simulink library "simulink"  (Simulink 6.0)
settings: Solver=ode45  SolverMode=SingleTasking  StartTime=0.0  StopTime=10.0  RelTol=1e-3
PostLoadFcn:
  | setsysloc(bdroot)
undefined symbols (not defined in the file or in its folder): DiscIntNeverNeededParam, getdatatypespecs, NumBits1, NumBits2, sfunxy, sigbuilder_block, slcm, Slope1, Slope2
libraries: simulink x82, eml_lib x1
(part 1 of 5)
settings Model: RequirementInfo=9  CovMetricSettings=d  Creator=ricks  LastModifiedBy=dyang  ExtModeAutoUpdateStatusClock=off  ProdHWDeviceType=Specified
settings Model: ForwardingTableString=|
  | ||__slOldName__||simulink/Discrete/Additional
  | Transfer Fcns/Weighted
  | Moving Average||__slNewName__||simulink/Discrete/Weighted
  | Moving Average||__slOldName__||simulink/Discrete/Additional
  | Transfer Fcns/Transfer Fcn
  | Direct Form I||__slNewName__||fixpt_lib_4/Filters/Filter
  | Direct Form I||__slOldName__||simulink/Bit
  | Operations/Bitwise
  | Operator||__slNewName__||simulink/Logic and Bit
  | Operations/Bitwise
  | Operator||__slOldName__||simulink/Logic and Bit
  | Operations/Bitwise
  | Logical Operator||__slNewName__||simulink/Logic and Bit
  | Operations/Bitwise
  | Operator||__slOldName__||simulink/Math
  | Operations/Bitwise
  | Logical Operator||__slNewName__||simulink/Logic and Bit
  | Operations/Bitwise
  | Operator||__slOldName__||simulink/Look-Up
  | Tables/Direct Look-Up
  | Table (n-D)||__slNewName__||simulink/Lookup
  | Tables/Direct Lookup
  | Table (n-D)||__slOldName__||simulink/Look-Up
  | Tables/Interpolation (n-D)
  | using PreLook-Up||__slNewName__||simulink/Lookup
  | Tables/Interpolation (n-D)
  | using PreLookup||__slOldName__||simulink/Look-Up
  | Tables/PreLook-Up
  | Index Search||__slNewName__||simulink/Lookup
  | Tables/PreLookup
  | Index Search||__slOldName__||simulink/Look-Up
  | Tables/Look-Up
  | Table (n-D)||__slNewName__||simulink/Lookup
  | Tables/Lookup
  | Table (n-D)||__slOldName__||simulink/Linear/Matrix
  | Gain||__slNewName__||simulink3/Math/Matrix
  | Gain||__slOldName__||simulink/Connections/Model Info||__slNewName__||simulink/Model-Wide
  | Utilities/Model Info||__slOldName__||simulink/Nonlinear/Manual Switch||__slNewName__||simulink/Signal
  | Routing/Manual Switch||__slOldName__||simulink/Nonlinear/Coulomb &
  | Viscous Friction||__slNewName__||simulink/Discontinuities/Coulomb &
  | Viscous Friction||__slOldName__||simulink/Linear/Slider
  | Gain||__slNewName__||simulink/Math
  | Operations/Slider
  | Gain||__slOldName__||simulink/Nonlinear/Algebraic Constraint||__slNewName__||simulink/Math
  | Operations/Algebraic Constraint||__slOldName__||simulink/Nonlinear/Look-Up
  | Table (2-D)||__slNewName__||simulink/Lookup
  | Tables/Lookup
  | Table (2-D)||__slOldName__||simulink/Linear/Dot Product||__slNewName__||simulink/Math
  | Operations/Dot Product
settings DataIOCC: SignalLoggingName=logsOut
settings OptimizationCC: BooleanDataType=off
settings DebuggingCC: CheckExecutionContextPreStartOutputMsg=on  CheckExecutionContextRuntimeOutputMsg=on  SolverPrmCheckMsg=none
settings HardwareCC: ProdHWDeviceType=Specified  TargetUnknown=on
settings ModelReferenceCC: UpdateModelReferenceTargets=IfOutOfDate

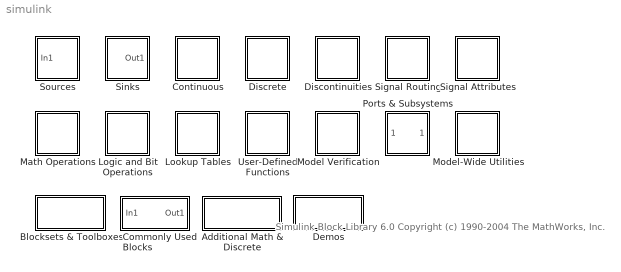
== system simulink ==
  note: Simulink Block Library 6.0
      | Copyright (c) 1990-2004
      | The MathWorks, Inc.
  Additional Math & Discrete : Subsystem
      mask Display: image(imread('additional_math_discrete.bmp','bmp'))
  Blocksets & Toolboxes : Subsystem
      settings: OpenFcn=findblib
      mask Display: image(imread('blocksets.bmp','bmp'))
  Commonly Used Blocks : Subsystem
      mask Display: image(imread('commonly_used.bmp','bmp'))
  Continuous : Subsystem
      mask Display: image(imread('continuous.bmp','bmp'))
  Demos : Subsystem
      settings: OpenFcn=demo simulink
      mask Display: image(imread('demos.bmp','bmp'))
  Discontinuities : Subsystem
      mask Display: image(imread('nonlinear.bmp','bmp'))
  Discrete : Subsystem
      mask Display: image(imread('discrete.bmp','bmp'))
  Logic and Bit Operations : Subsystem
      mask Display: image(imread('logical_bit.bmp','bmp'))
  Lookup Tables : Subsystem
      mask Display: image(imread('tables.bmp','bmp'))
  Math Operations : Subsystem
      mask Display: image(imread('math.bmp','bmp'))
  Model Verification : Subsystem
      mask Display: image(imread('assertion.bmp','bmp'))
  Model-Wide Utilities : Subsystem
      mask Display: image(imread('misc.bmp','bmp'))
  Ports & Subsystems : Subsystem  TreatAsAtomicUnit=on
      mask Display: image(imread('subsystems.bmp','bmp'))
  Signal Attributes : Subsystem
      mask Display: image(imread('attributes.bmp','bmp'))
  Signal Routing : Subsystem
      mask Display: image(imread('signals.bmp','bmp'))
  Sinks : Subsystem
      mask Display: image(imread('sinks.bmp','bmp'))
  Sources : Subsystem
      mask Display: image(imread('sources.bmp','bmp'))
  User-Defined Functions : Subsystem
      mask Display: image(imread('functions.bmp','bmp'))

== system simulink/Additional Math & Discrete ==
  note: Additional Math & Discrete
  Additional Discrete : Subsystem
      mask Display: image(imread('discrete.bmp','bmp'))
  Additional Math: Increment - Decrement : Subsystem
      mask Display: image(imread('increment_decrement.bmp','bmp'))

== system simulink/Blocksets & Toolboxes ==

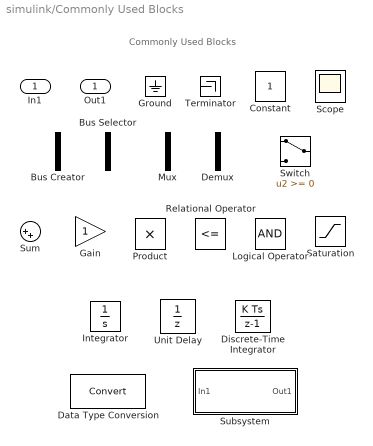
== system simulink/Commonly Used Blocks ==
  note: Commonly Used Blocks
  In1 : Inport  LatchInput=off
  Bus Creator : BusCreator  DialogController=Simulink.DDGSource_Bus  Inputs=2
      settings: CopyFcn=set_param(gcbh,'ShowName','off','CopyFcn','')
  Bus Selector : BusSelector  DialogController=Simulink.DDGSource_Bus  OutputSignals=signal1,signal2
      settings: CopyFcn=set_param(gcbh,'ShowName','off','CopyFcn','')
  Constant : Constant
  Data Type Conversion : DataTypeConversion
  Demux : Demux  Outputs=2
      settings: CopyFcn=set_param(gcbh,'ShowName','off','CopyFcn','')
  Discrete-Time Integrator : DiscreteIntegrator  ICPrevOutput=DiscIntNeverNeededParam  ICPrevScaledInput=DiscIntNeverNeededParam
  Gain : Gain
  Ground : Ground
  Integrator : Integrator
  Logical Operator : Logic  AllPortsSameDT=off  OutDataTypeMode=Boolean
  Mux : Mux  Inputs=2
      settings: CopyFcn=set_param(gcbh,'ShowName','off','CopyFcn','')
  Product : Product  RndMeth=Zero
  Relational Operator : RelationalOperator  Operator=<=  LogicOutDataTypeMode=Boolean
  Saturation : Saturate
  Scope : Scope
      settings: SaveName=ScopeData2
  Subsystem : Subsystem
      settings: CopyFcn=set_param(gcbh,'LinkStatus','none'); set_param(gcbh,'Mask','off'); set_param(gcbh,'MaskType',''); set_param(gcbh,'MaskDescription',''); set_param(gcbh,'OpenFcn',''); set_param(gcbh,'CopyFcn','')  OpenFcn=open_system(gcbh,'force')
      mask Type: Virtual Subsystem
      mask Description: A subsystem block template containing an inport and outport block.
  Sum : Sum  Inputs=|++
      settings: CopyFcn=set_param(gcbh,'ShowName','off','CopyFcn','')
  Switch : Switch
  Terminator : Terminator
  Unit Delay : UnitDelay
  Out1 : Outport

== system simulink/Continuous ==
  note: Continuous-Time Linear Systems
  note: Continuous-Time Delays
  Derivative : Derivative
  Integrator : Integrator
  State-Space : StateSpace
  Transfer Fcn : TransferFcn  Denominator=[1 1]
  Transport Delay : TransportDelay
  Variable Transport Delay : VariableTransportDelay  MaximumDelay=10
  Zero-Pole : ZeroPole  Poles=[0 -1]

== system simulink/Demos ==

== system simulink/Discontinuities ==
  note: Discontinuities
  Backlash : Backlash
  Coulomb & Viscous Friction : Subsystem  mask(Coulombic and Viscous Friction){offset=[1 3 2 0], gain=1}
      mask prompts: offset "Coulomb friction value (Offset):"; gain "Coefficient of viscous friction (Gain):"
      mask help:
      | A discontinuity offset at zero models coulomb friction.  Linear gain models viscous friction.
      | y = sign(x) * (Gain * abs(x) + Offset)
      mask init:
      | x=max(offset(1),gain(1)+offset(1));
      mask Help:
      | This block has a discontinuity
      | at zero and a linear gain afterward.
      | y= sign(x)*(Gain*abs(x)+Offset)
      mask Display: plot([-1 0 0 1],[-gain(1)-offset(1), -offset(1), offset(1), gain(1)+offset(1)],[-1 1],[0 0],[0 0],[-x,x])
  Dead Zone : DeadZone  SaturateOnIntegerOverflow=on
  Dead Zone Dynamic : Subsystem
      mask Type: Dead Zone Dynamic
      mask Description: Output zero for inputs within deadzone.  Offset input signals by either the Start or End value when outside of the deadzone.
      mask Display: plot([0.15 0.85],[.5 .5],[.5 .5],[0.05 0.95],0.15+0.7*[0 .3 .7 1],0.05+0.9*[0.1 0.5 0.5 0.9]);
  Hit  Crossing : HitCross
  Quantizer : Quantizer
  Rate Limiter : RateLimiter  SampleTimeMode=inherited
  Rate Limiter Dynamic : Subsystem
      mask Type: Rate Limiter Dynamic
      mask Description: Limit rising and falling rates of the signals at the second input by using the first input (upper limit) and the third input (lower limit).
      mask Display: plot([0.15 0.95],[.5 .5],[.5 .5],[0.05 0.95],0.05+0.9*[.2 .8],0.05+0.9*[0 1]);
  Relay : Relay
  Saturation : Saturate
  Saturation Dynamic : Subsystem
      mask Type: Saturation Dynamic
      mask Description: Bound the range of the second input by using the first input (upper limit) and the third input (lower limit).
      mask Display: plot([0.15 0.85],[.5 .5],[.5 .5],[0.05 0.95],0.15+0.7*[0 .25 .75 1],0.05+0.9*[.25 .25 .75 .75]);
  Wrap To Zero : Subsystem  mask(Wrap To Zero){Threshold=255}
      mask help: If the input is above the threshold, the output is zero, otherwise the output equals the input.
      mask Display: plot([0.1 0.9],[.3 .3],[.2 .2],[0.2 0.9],[0.1 .7 .7 .9],[0.2 0.8 .325 .325],0.05+[0.1 0.2 NaN 0.3 0.4 NaN 0.5 0.6 NaN 0.7 0.8],0.8*ones(1,11));

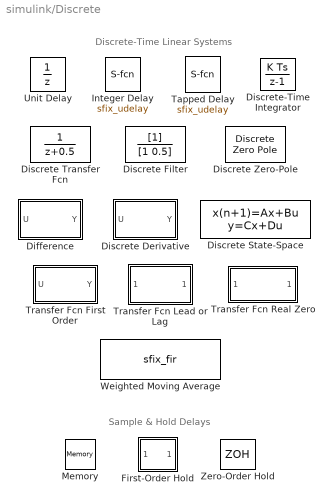
== system simulink/Discrete ==
  note: Sample & Hold Delays
  note: Discrete-Time Linear Systems
  Difference : Subsystem  mask(Difference){ICPrevInput=0.0, OutputDataTypeScalingMode=Inherit via internal rule, OutDataType=sfix(16), OutScaling=2^-10, LockScale=off, RndMeth=Floor, DoSatur=off}
      mask prompts: ICPrevInput "Initial condition for previous input:"; OutputDataTypeScalingMode "Output data type and scaling:"; OutDataType "Output data type:     ex.  sfix(16),  uint(8),  float('single')"; OutScaling "Output scaling:    Slope or [Slope Bias]    ex.  2^-9"; LockScale "Lock output scaling so autoscaling tool can't change it"; RndMeth "Round toward:"; DoSatur "Saturate to max or min when overflows occur"
      mask help: Output the current input value minus the previous input value.
      mask init:
      | blkH = gcbh;
      | blkName = getfullname(blkH);
      | 
      | switch OutputDataTypeScalingMode
      |   case 1
      |     diffMode   = 'Specify via dialog';
      |   case 2
      |     diffMode   = 'Inherit via internal rule';
      |   otherwise
      |     diffMode   = 'Inherit via back propagation';
      | end
      | vRndMeth = get_param(blkH,'RndMeth');
      | vDoSatur = get_param(blkH,'DoSatur');
      | set_param([blkName,'/Diff'],'OutputDataTypeScalingMode',  diffMode, ...
      | 	'RndMeth',vRndMeth, ...
      | 	'DoSatur',vDoSatur);
      mask StyleString: edit,popup(Specify via dialog|Inherit via internal rule|Inherit via back propagation),edit,edit,checkbox,popup(Zero|Nearest|Ceiling|Floor),checkbox
      mask CallbackString: |fixptdialog(gcbh)|fixptdialog(gcbh)||||
      mask TabNameString: Main,Signal data types,Signal data types,Signal data types,Signal data types,Signal data types,Signal data types
      mask Display: dpoly([1 -1],[1 0],'z')
  Discrete Transfer Fcn : DiscreteTransferFcn
  Discrete Zero-Pole : DiscreteZeroPole  Poles=[0 0.5]  Gain=1
  Discrete Derivative : Subsystem  mask(Discrete Derivative){gainval=1.0, ICPrevScaledInput=0.0, OutputDataTypeScalingMode=Inherit via internal rule, OutDataType=sfix(16), OutScaling=2^-10, LockScale=off, RndMeth=Floor, DoSatur=off}
      mask prompts: gainval "Gain value:"; ICPrevScaledInput "Initial condition for previous weighted input K*u/Ts:"; OutputDataTypeScalingMode "Output data type and scaling:"; OutDataType "Output data type:     ex.  sfix(16),  uint(8),  float('single')"; OutScaling "Output scaling:    Slope or [Slope Bias]    ex.  2^-9"; LockScale "Lock output scaling so autoscaling tool can't change it"; RndMeth "Round toward:"; DoSatur "Saturate to max or min when overflows occur"
      mask help:
      | Discrete-time derivative of the input.
      |
      | This block only works with fixed sample rates, so it will not work inside a triggered subsystem.
      mask init:
      | blkH = gcbh;
      | blkName = getfullname(blkH);
      | 
      | switch OutputDataTypeScalingMode
      |   case 1
      |     diffMode   = 'Specify via dialog';
      |     tsampMode  = 'Inherit via back propagation';
      |     tsampImp  = 'Online Calculations';
      |   case 2
      |     diffMode   = 'Inherit via back propagation';
      |     tsampMode  = 'Inherit via internal rule';
      |     tsampImp  = 'Offline Scaling Adjustment';
      |   otherwise
      |     diffMode   = 'Inherit via back propagation';
      |     tsampMode  = 'Inherit via back propagation';
      |     tsampImp  = 'Online Calculations';
      | end
      | vRndMeth = get_param(blkH,'RndMeth');
      | vDoSatur = get_param(blkH,'DoSatur');
      | set_param([blkName,'/Diff'],'OutputDataTypeScalingMode',  diffMode, ...
      | 	'RndMeth',vRndMeth, ...
      | 	'DoSatur',vDoSatur);
      | set_param([blkName,'/TSamp'],'TsampMathImp',tsampImp,'OutputDataTypeScalingMode',tsampMode, ...
      | 	'RndMeth',vRndMeth, ...
      | 	'DoSatur',vDoSatur);
      mask StyleString: edit,edit,popup(Specify via dialog|Inherit via internal rule|Inherit via back propagation),edit,edit,checkbox,popup(Zero|Nearest|Ceiling|Floor),checkbox
      mask CallbackString: ||fixptdialog(gcbh)|fixptdialog(gcbh)||||
      mask TabNameString: Main,Main,Signal data types,Signal data types,Signal data types,Signal data types,Signal data types,Signal data types
      mask Display: text(0.5, 0.5, 'K (z-1)', 'horizontalAlignment', 'center', 'verticalAlignment', 'bottom');text(0.5, 0.5, 'Ts z', 'horizontalAlignment', 'center', 'verticalAlignment', 'top');plot([0.3 0.7],[0.5 0.5]);
  Discrete Filter : DiscreteFilter  Denominator=[1 0.5]
  Discrete State-Space : DiscreteStateSpace
  Discrete-Time Integrator : DiscreteIntegrator  ICPrevOutput=DiscIntNeverNeededParam  ICPrevScaledInput=DiscIntNeverNeededParam
  First-Order Hold : Subsystem  DisableCoverage=on  mask(First-Order Hold){Ts=1}
      mask prompts: Ts "Sample time:"
      mask help: First-order hold.
      mask Help: This block implements a first-order hold by extrapolating between sample points using a first-order polynomial.
      mask Display: plot(0,0,100,100,[90,70,50,30,10],[60,40,80,30,20])
  Integer Delay : S-Function  FunctionName=sfix_udelay  Parameters=samptime,vinit,NumDelays,1,1,0  mask(Integer Delay){vinit=0.0, samptime=-1, NumDelays=4}
      mask prompts: vinit "Initial condition:"; samptime "Sample time:"; NumDelays "Number of delays:"
      mask help: Delay a signal N sample periods.
      mask init:
      | if isempty(NumDelays)
      |    NumDelays = 1;
      | end
      mask Display: fprintf(' %d\nZ   ',-1*(NumDelays))
  Memory : Memory
  Tapped Delay : S-Function  FunctionName=sfix_udelay  Parameters=samptime,vinit,NumDelays,NumDelays,DelayOrder,includeCurrent  mask(Tapped Delay Line){vinit=0.0, samptime=-1, NumDelays=4, DelayOrder=Oldest, includeCurrent=off}
      mask prompts: vinit "Initial condition:"; samptime "Sample time:"; NumDelays "Number of delays:"; DelayOrder "Order output vector starting with:"; includeCurrent "Include current input in output vector"
      mask help: Delay a signal N sample periods and output all the delay versions.
      mask init:
      | if isempty(NumDelays)
      |    NumDelays = 1;
      | end
      mask StyleString: edit,edit,edit,popup(Oldest|Newest),checkbox
      mask Display: fprintf(' %d\nDelays\n',(NumDelays))
  Transfer Fcn First Order : Subsystem  mask(First Order Transfer Fcn){PoleZ=0.95, ICPrevOutput=0.0, RndMeth=Floor, DoSatur=off}
      mask prompts: PoleZ "Pole (in Z plane):"; ICPrevOutput "Initial condition for previous output:"; RndMeth "Round toward:"; DoSatur "Saturate to max or min when overflows occur"
      mask help: Discrete-time first order transfer function. The transfer function has a unity DC gain.
      mask init:
      | blkH = gcbh;
      | blkName = getfullname(blkH);
      | 
      | vRndMeth = get_param(blkH,'RndMeth');
      | vDoSatur = get_param(blkH,'DoSatur');
      | 
      | set_param([blkName,'/Gain'],'RndMeth',vRndMeth, ...
      | 	'DoSatur',vDoSatur);
      | set_param([blkName,'/Diff'],'RndMeth',vRndMeth, ...
      | 	'DoSatur',vDoSatur);
      | set_param([blkName,'/Sum'],'RndMeth',vRndMeth, ...
      | 	'DoSatur',vDoSatur);
      mask StyleString: edit,edit,popup(Zero|Nearest|Ceiling|Floor),checkbox
      mask Display: dpoly([1-PoleZ 0],[1 -PoleZ],'z')
  Transfer Fcn Lead or Lag : Subsystem  mask(Lead or Lag Compensator){PoleZ=0.95, ZeroZ=0.75, ICPrevOutput=0.0, ICPrevInput=0.0, RndMeth=Floor, DoSatur=off}
      mask prompts: PoleZ "Pole of compensator (in Z plane):"; ZeroZ "Zero of compensator (in Z plane):"; ICPrevOutput "Initial condition for previous output:"; ICPrevInput "Initial condition for previous input:"; RndMeth "Round toward:"; DoSatur "Saturate to max or min when overflows occur"
      mask help:
      | Discrete-time lead or lag compensator.  The compensator has a unity instantaneous gain, the DC gain equals (1-Zero)/(1-Pole).
      |
      | Lead compensation is obtained when 0 < Pole < Zero < 1.
      | Lag compensation is obtained when 0 < Zero < Pole < 1.
      mask init:
      | blkH = gcbh;
      | blkName = getfullname(blkH);
      | 
      | vRndMeth = get_param(blkH,'RndMeth');
      | vDoSatur = get_param(blkH,'DoSatur');
      | DCGain = (1-ZeroZ)./(1-PoleZ);
      | maxGain = max( 1, max(max(abs(DCGain))) );
      | OutputSlopeMult = 2^ceil(log2(maxGain));
      | set_param([blkName,'/GainZero'],'RndMeth',vRndMeth, ...
      | 	'DoSatur',vDoSatur);
      | set_param([blkName,'/GainPole'],'RndMeth',vRndMeth, ...
      | 	'DoSatur',vDoSatur);
      | set_param([blkName,'/Downcast'],'RndMeth',vRndMeth, ...
      | 	'DoSatur',vDoSatur);
      | set_param([blkName,'/Sum'],'RndMeth',vRndMeth, ...
      | 	'DoSatur',vDoSatur);
      mask StyleString: edit,edit,edit,edit,popup(Zero|Nearest|Ceiling|Floor),checkbox
      mask Display: dpoly([1 -ZeroZ],[1 -PoleZ],'z')
  Transfer Fcn Real Zero : Subsystem  mask(Transfer Fcn Real Zero){ZeroZ=0.75, ICPrevInput=0.0, RndMeth=Floor, DoSatur=off}
      mask prompts: ZeroZ "Zero (in Z plane):"; ICPrevInput "Initial condition for previous input:"; RndMeth "Round toward:"; DoSatur "Saturate to max or min when overflows occur"
      mask help: Discrete-time transfer function that has a real zero and (effectively) has no pole.
      mask init:
      | blkH = gcbh;
      | blkName = getfullname(blkH);
      | 
      | vRndMeth = get_param(blkH,'RndMeth');
      | vDoSatur = get_param(blkH,'DoSatur');
      | DCGain = (1-ZeroZ);
      | maxGain = max( 1, max(max(abs(DCGain))) );
      | OutputSlopeMult = 2^ceil(log2(maxGain));
      | set_param([blkName,'/GainZero'],'RndMeth',vRndMeth, ...
      | 	'DoSatur',vDoSatur);
      | set_param([blkName,'/Sum'],'RndMeth',vRndMeth, ...
      | 	'DoSatur',vDoSatur);
      mask StyleString: edit,edit,popup(Zero|Nearest|Ceiling|Floor),checkbox
      mask Display: dpoly([1 -ZeroZ],[1 0],'z')
  Unit Delay : UnitDelay
  Weighted Moving Average : S-Function  FunctionName=sfix_fir  Parameters=(getdatatypespecs(OutDataType,OutScaling,DblOver,0)),[DoSatur RndMeth-1],DblOver,dolog,mgainval,(getdatatypespecs(GainDataType,GainScaling,DblOver,RadixGroup)),samptime,vinit,OutputDataTypeScalingMode,GainDataTypeScalingMode  mask(Weighted Moving Average){mgainval=[0.1:0.1:1 0.9:-0.1:0.1], vinit=0.0, samptime=-1, GainDataTypeScalingMode=Inherit via internal rule, GainDataType=sfix( 16 ), MatRadixGroup=Best Precision: Matrix-wise, GainScaling=2^-10, OutputDataTypeScalingMode=Inherit via internal rule, OutDataType=sfix(16), OutScaling=2^-10, LockScale=off, RndMeth=Floor, DoSatur=off}
      mask prompts: mgainval "Weights:"; vinit "Initial condition:"; samptime "Sample time:"; GainDataTypeScalingMode "Gain data type and scaling:"; GainDataType "Parameter data type:     ex. sfix(16),  uint(8), float('single')"; MatRadixGroup "Parameter scaling mode:"; GainScaling "Parameter scaling:    Slope    ex.  2^-9"; OutputDataTypeScalingMode "Output data type and scaling:"; OutDataType "Output data type:     ex.  sfix(16),  uint(8),  float('single')"; OutScaling "Output scaling:    Slope or [Slope Bias]    ex.  2^-9"; LockScale "Lock output scaling so autoscaling tool can't change it"; RndMeth "Round toward:"; DoSatur "Saturate to max or min when overflows occur"
      mask help: Output the weighted moving average of the input.
      mask init:
      | DblOver = 0;
      | dolog = 0;
      | 
      | if MatRadixGroup == 5
      |     RadixGroup = 1; % BEST_PREC_MAT
      | elseif MatRadixGroup == 4
      |     RadixGroup = 2; % BEST_PREC_COL
      | elseif MatRadixGroup == 3
      |     RadixGroup = 3; % BEST_PREC_ROW
      | elseif MatRadixGroup == 2
      |     RadixGroup = 4; % BEST_PREC_ELE
      | else
      |     RadixGroup = 0; % BEST_PREC_OFF
      | end
      mask StyleString: edit,edit,edit,popup(Specify via dialog|Inherit via internal rule),edit,popup(Use Specified Scaling|Best Precision: Element-wise|Best Precision: Row-wise|Best Precision: Column-wise|Best Precision: Matrix-wise),edit,popup(Specify via dialog|Inherit via internal rule|Inherit via back propagation),edit,edit,checkbox,popup(Zero|Nearest|Ceiling|Floor),checkbox
      mask CallbackString: |||fixptdialog(gcbh)|fixptdialog(gcbh)|fixptdialog(gcbh)||fixptdialog(gcbh)|fixptdialog(gcbh)||||
      mask TabNameString: Main,Main,Main,Parameter data types,Parameter data types,Parameter data types,Parameter data types,Signal data types,Signal data types,Signal data types,Signal data types,Signal data types,Signal data types
      mask Display:
      | fprintf(fixpt_fir_mask_data(mgainval,'dispstr'))
      | plot(fixpt_fir_mask_data(mgainval,1),fixpt_fir_mask_data(mgainval,0))
  Zero-Order Hold : ZeroOrderHold

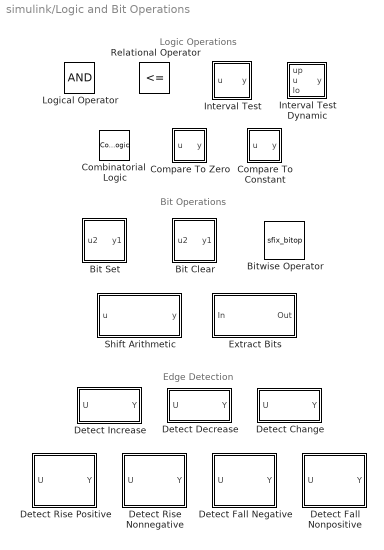
== system simulink/Logic and Bit Operations ==
  note: Edge Detection
  note: Logic Operations
  note: Bit Operations
  Bit Clear : Subsystem  mask(Bit Clear){iBit=0}
      mask prompts: iBit "Index of bit (0 is least significant):"
      mask help: Clear ith bit of the stored integer to 0. Scaling is ignored.
      mask Display: fprintf('Clear\nbit %d',iBit)
  Bit Set : Subsystem  mask(Bit Set){iBit=0}
      mask prompts: iBit "Index of bit (0 is least significant):"
      mask help: Set ith bit of the stored integer to 1. Scaling is ignored.
      mask Display: fprintf('Set\nbit %d',iBit)
  Bitwise Operator : S-Function  FunctionName=sfix_bitop  Parameters=UseBitMask,NumInputPorts,BitMask,BitMaskRealWorld,logicop  mask(Bitwise Operator){logicop=AND, UseBitMask=on, NumInputPorts=1, BitMask=bin2dec('11011001'), BitMaskRealWorld=Stored Integer}
      mask prompts: logicop "Operator:"; UseBitMask "Use bit mask ..."; NumInputPorts "Number of input ports:"; BitMask "Bit Mask"; BitMaskRealWorld "Treat mask as:"
      mask help: Perform the specified bitwise operation on the inputs. The output data type should represent zero exactly.
      mask init:
      | if UseBitMask
      |   [m,n] = size(BitMask);
      |   if ischar(BitMask)
      |     len = m;
      |     n = 1;
      |   else
      |     len = m * n;
      |   end
      |   internalBitMask = zeros(m,n);
      |   if isnumeric(BitMask)
      |     for i=1:len,
      |       internalBitMask(i) = BitMask(i);
      |     end
      |   elseif ischar(BitMask)
      |     for i=1:m,
      |       internalBitMask(i) = hex2dec(BitMask(i,:));
      |     end
      |   elseif iscell(BitMask)
      |     for i=1:len,
      |       if isnumeric( BitMask{i} )
      |         internalBitMask(i) = BitMask{i};
      |       elseif ischar( BitMask{i} )
      |         internalBitMask(i) = hex2dec(BitMask{i});
      |       else
      |         errordlg(['Data type is not supported at cell item ', num2str(i) ]);
      |       end
      |     end
      |   end
      |   if BitMaskRealWorld == 1
      |      BitMask = internalBitMask;
      |   else
      |      BitMask = fix(internalBitMask);
      |   end
      |   if len == 1
      |      if BitMaskRealWorld == 1
      |        str=num2str(BitMask(1));
      |      else
      |        str=['0x',dec2hex(BitMask(1))];
      |      end
      |   else
      |      str='Masks';
      |   end
      | else
      |   BitMask = 0;
      |   str='';
      | end
      mask StyleString: popup(AND|OR|NAND|NOR|XOR|NOT),checkbox,edit,edit,popup(Real World Value|Stored Integer)
      mask CallbackString: fixptdialog(gcbh)|fixptdialog(gcbh)|||
      mask Display: fprintf(['Bitwise\n',logicop,'\n',str])
  Combinatorial  Logic : CombinatorialLogic
  Compare To Constant : Subsystem  mask(Compare To Constant){relop=<=, const=3.0, LogicOutDataTypeMode=uint8}
      mask prompts: relop "Operator:"; const "Constant value:"; LogicOutDataTypeMode "Output data type mode:"
      mask help: Determine how a signal compares to a constant.
      mask init:
      | blkName = gcb;
      | 
      | if strcmp(get_param(gcbh,'LogicOutDataTypeMode'),'boolean')
      | 	setValue = 'Boolean';
      | else
      | 	setValue = 'Specify via dialog';
      | end
      | 
      | set_param([blkName,'/Compare'],'relop',relop, ...
      | 	'LogicOutDataTypeMode', setValue);
      | 
      | if length(const) == 1
      |  str = [relop,' ',num2str(double(const))];
      | else
      |   str = [relop,' C'];
      | end
      mask StyleString: popup(==|~=|<|<=|>=|>),edit,popup(uint8|boolean)
      mask Display: disp(str)
  Compare To Zero : Subsystem  mask(Compare To Zero){relop=<=, LogicOutDataTypeMode=uint8}
      mask prompts: relop "Operator:"; LogicOutDataTypeMode "Output data type mode:"
      mask help: Determine how a signal compares to zero.
      mask init:
      | blkName = gcb;
      | 
      | if strcmp(get_param(gcbh,'LogicOutDataTypeMode'),'boolean')
      | 	setValue = 'Boolean';
      | else
      |     setValue = 'Specify via dialog';
      | end
      | 
      | set_param([blkName,'/Compare'],'relop',relop, ...
      | 	'LogicOutDataTypeMode', setValue);
      mask StyleString: popup(==|~=|<|<=|>=|>),popup(uint8|boolean)
      mask Display: disp([relop,' 0'])
  Detect Change : Subsystem  mask(Detect Change){vinit=0}
      mask prompts: vinit "Initial condition:"
      mask help: If the input does not equal its previous value, then output TRUE, otherwise output FALSE. The initial condition determines the initial value of the previous input U/z.
      mask Display: fprintf('U ~= U/z')
  Detect Decrease : Subsystem  mask(Detect Decrease){vinit=0.0}
      mask prompts: vinit "Initial condition:"
      mask help: If the input is strictly less than its previous value, then output TRUE, otherwise output FALSE. The initial condition determines the initial value of the previous input U/z.
      mask Display: fprintf('U < U/z')
  Detect Increase : Subsystem  mask(Detect Increase){vinit=0.0}
      mask prompts: vinit "Initial condition:"
      mask help: If the input is strictly greater than its previous value, then output TRUE, otherwise output FALSE. The initial condition determines the initial value of the previous input U/z.
      mask Display: fprintf('U > U/z')
  Detect Fall Negative : Subsystem  mask(Detect Fall Negative){vinit=0}
      mask prompts: vinit "Initial condition:"
      mask help: If the input is strictly negative and its previous value was nonnegative, then output TRUE, otherwise output FALSE. The initial condition determines the initial value of the boolean expression (U/z < 0).
      mask init:
      | vinit=double(vinit);
      mask Display: fprintf('U < 0\n&  NOT\nU/z < 0')
  Detect Fall Nonpositive : Subsystem  mask(Detect Fall Nonpositive){vinit=0}
      mask prompts: vinit "Initial condition:"
      mask help: If the input is nonpositive and its previous value was strictly positive, then output TRUE, otherwise output FALSE. The initial condition determines the initial value of the boolean expression (U/z <= 0).
      mask init:
      | vinit=double(vinit);
      mask Display: fprintf('U <= 0\n&  NOT\nU/z <= 0')
  Detect Rise Nonnegative : Subsystem  mask(Detect Rise Nonnegative){vinit=0}
      mask prompts: vinit "Initial condition:"
      mask help: If the input is nonnegative and its previous value was strictly negative, then output TRUE, otherwise output FALSE. The initial condition determines the initial value of the boolean expression (U/z >= 0).
      mask init:
      | vinit=double(vinit);
      mask Display: fprintf('U >= 0\n&  NOT\nU/z >= 0')
  Detect Rise Positive : Subsystem  mask(Detect Rise Positive){vinit=0}
      mask prompts: vinit "Initial condition:"
      mask help: If the input is strictly positive and its previous value was nonpositive, then output TRUE, otherwise output FALSE. The initial condition determines the initial value of the boolean expression (U/z > 0).
      mask init:
      | vinit=double(vinit);
      mask Display: fprintf('U > 0\n&  NOT\nU/z > 0')
  Extract Bits : Subsystem  mask(Extract Bits){bitsToExtract=Upper half, numBits=8, bitIdxRange=[0 7], outScalingMode=Preserve fixed-point scaling}
      mask prompts: bitsToExtract "Bits to extract:"; numBits "Number of bits:"; bitIdxRange "Bit indices ([start end], 0-based relative to LSB):"; outScalingMode "Output scaling mode:"
      mask help: Output selected bits from each of the fixed-point input samples. Selecting "Upper half" or "Lower half" results in a positive number of bits in the output word length, according to the equation numOutputBits = ceil(numInputBits / 2).
      mask init:
      | str = fixpt_extractbits_mask('icon'); 
      | fixpt_extractbits_mask_script;
      mask StyleString: popup(Upper half|Lower half|Range starting with most significant bit|Range ending with least significant bit|Range of bits),edit,edit,popup(Preserve fixed-point scaling|Treat bit field as an integer)
      mask CallbackString: fixpt_extractbits_mask;|||
      mask Display: disp(str);
  Interval Test : Subsystem  mask(Interval Test){IntervalClosedRight=on, uplimit=0.5, IntervalClosedLeft=on, lowlimit=-0.5, LogicOutDataTypeMode=boolean}
      mask prompts: IntervalClosedRight "Interval closed on right"; uplimit "Upper limit:"; IntervalClosedLeft "Interval closed on left"; lowlimit "Lower limit:"; LogicOutDataTypeMode "Output data type mode:"
      mask help: If the input is in the interval between the lower limit and the upper limit, then the output is TRUE, otherwise it is FALSE.
      mask init:
      | if IntervalClosedLeft
      |   lOff = 0;
      |   lRelop = '<=';
      | else
      |   lOff = 0.1;
      |   lRelop = '<';
      | end
      | if IntervalClosedRight
      |   rOff = 0;
      |   uRelop = '<=';
      | else
      |   rOff = 0.1;
      |   uRelop = '<';
      | end
      | 
      | blkH = gcbh;
      | blkName = getfullname(blkH);
      | 
      | set_param([blkName,'/Upper Test'],'relop',uRelop);
      | set_param([blkName,'/Lower Test'],'relop',lRelop);
      | if strcmp(get_param(blkH,'LogicOutDataTypeMode'),'boolean')
      | set_param([blkName,'/AND'],'OutDataTypeMode','Boolean');
      | else
      | set_param([blkName,'/AND'],'OutDataTypeMode','Specify via dialog');
      | end
      mask StyleString: checkbox,edit,checkbox,edit,popup(uint8|boolean)
      mask Display: plot([0 1],[0.3 0.3],[0.3 0.3],[0 1],[0 0.2 0.2],[0.35 0.35 0.55-lOff],[0.2 0.2 0.55 0.55],[0.55+lOff 0.75 0.75 0.55+rOff],[0.55 0.55 1],[0.55-rOff 0.35 0.35]);
  Interval Test Dynamic : Subsystem  mask(Interval Test Dynamic){IntervalClosedRight=on, IntervalClosedLeft=on, LogicOutDataTypeMode=boolean}
      mask prompts: IntervalClosedRight "Interval closed on right"; IntervalClosedLeft "Interval closed on left"; LogicOutDataTypeMode "Output data type mode:"
      mask help: If the input is in the interval between the lower limit and the upper limit, then the output is TRUE, otherwise it is FALSE.
      mask init:
      | if IntervalClosedLeft
      |   lOff = 0;
      |   lRelop = '<=';
      | else
      |   lOff = 0.1;
      |   lRelop = '<';
      | end
      | if IntervalClosedRight
      |   rOff = 0;
      |   uRelop = '<=';
      | else
      |   rOff = 0.1;
      |   uRelop = '<';
      | end
      | blkH = gcbh;
      | blkName = getfullname(gcbh);
      | 
      | set_param([blkName,'/Upper Test'],'relop',uRelop);
      | set_param([blkName,'/Lower Test'],'relop',lRelop);
      | if strcmp(get_param(blkH,'LogicOutDataTypeMode'),'boolean')
      | set_param([blkName,'/FixPt Logical Operator'],'OutDataTypeMode','Boolean');
      | else
      | set_param([blkName,'/FixPt Logical Operator'],'OutDataTypeMode','Specify via dialog');
      | end
      mask StyleString: checkbox,checkbox,popup(uint8|boolean)
      mask Display: plot(0.35+0.65*[0 1],[0.3 0.3],0.35+0.65*[0.3 0.3],[0 1],0.35+0.65*[0 0.2 0.2],[0.35 0.35 0.55-lOff],0.35+0.65*[0.2 0.2 0.55 0.55],[0.55+lOff 0.75 0.75 0.55+rOff],0.35+0.65*[0.55 0.55 1],[0.55-rOff 0.35 0.35]);
  Logical Operator : Logic  AllPortsSameDT=off  OutDataTypeMode=Boolean
  Relational Operator : RelationalOperator  Operator=<=  LogicOutDataTypeMode=Boolean
  Shift Arithmetic : Subsystem  mask(Shift Arithmetic){nBitShiftRight=8, nBinPtShiftRight=0}
      mask prompts: nBitShiftRight "Number of bits to shift right (use negative value to shift left):"; nBinPtShiftRight "Number of places by which binary point shifts right (use negative value to shift left):"
      mask help:
      | This block can arithmetically shift the bits and/or the binary point of a signal.
      | The effect of these actions can be interpreted as a combination of a multiplication by a power of two and a change in scaling.  The power of two multiplication term is
      |   2^( NumBinaryPointShiftsRight - NumBitShiftsRight )
      | Negative values for shifts right are actually positive shift lefts.
      | If the input is a floating point type, the power of two multiplication is carried out, but no change in scaling is applied.
      mask init:
      | netExponent = nBinPtShiftRight - nBitShiftRight;
      | netExponent(find(netExponent>127)) = 127;
      | netExponent(find(netExponent<-127)) = -127;
      | nBitShiftRight(find(nBitShiftRight>127)) = 127;
      | nBitShiftRight(find(nBitShiftRight<-127)) = -127;
      | dstr = ['Vy = Vu'];
      | if netExponent ~= 0
      |   dstr = [dstr,' * 2^',num2str(netExponent)];
      | end
      | dstr = [dstr,'\nQy = Qu'];
      | if nBitShiftRight > 0
      |   dstr = [dstr,' >> ',num2str(nBitShiftRight)];
      | elseif nBitShiftRight < 0
      |  dstr = [dstr,' << ',num2str(-nBitShiftRight)];
      | end
      | dstr = [dstr,'\nEy = Eu'];
      | if nBinPtShiftRight > 0
      |   dstr = [dstr,' + ',num2str(nBinPtShiftRight)];
      | elseif nBinPtShiftRight < 0
      |   dstr = [dstr,' - ',num2str(-nBinPtShiftRight)];
      | end
      | for i = 1:length(netExponent)
      |     netExponent(i) = 2^netExponent(i);
      | end
      mask Display: fprintf(dstr)

== system simulink/Lookup Tables ==
  note: Lookup Tables
  Cosine : Subsystem  mask(Cosine){NumDataPoints=(2^5)+1}
      mask prompts: NumDataPoints "Number of data points for lookup table:"
      mask help:
      | Implement a Cosine function in Fixed-Point using a lookup table approach that exploits quarter wave symmetry.  The output is normally a signed 16 bit number with 14 bits to the right of the binary point.
      |
      | The most efficient implementation is obtained when the number of data points is a power of 2 plus 1.  For example, (2^5)+1.
      mask init:
      | XData = linspace(0,0.25,NumDataPoints);
      | %
      | % using sin for the data is not a mistake.
      | % parameter pooling will cause the data for similar sines and cosines to
      | % be shared.  This can save significant amounts of ROM.
      | %
      | YData = sin(2*pi*XData);
      mask Display: disp('cos(2*pi*u)')
  Direct Lookup Table (n-D) : S-Function  FunctionName=sfun_nddirectlook  Parameters=numInputs,mxTable,clipFlag,tabIsInput,numTDims  mask(LookupNDDirect){maskTabDims=2, explicitNumDims=1, outDims=Element, tabIsInput=off, mxTable=[4 5 6;16 19 20;10 18 23], clipFlag=Warning}
      mask prompts: maskTabDims "Number of table dimensions:"; explicitNumDims "Explicit number of table dimensions:"; outDims "Inputs select this object from table:"; tabIsInput "Make table an input"; mxTable "Table data:"; clipFlag "Action for out of range input:"
      mask help: Table member selection. Inputs are zero-based indices into the table, e.g., an input of 3 returns the fourth element in that dimension. Block can also be used to select a column or 2-D matrix out of the table. The first selection index corresponds to the top (or left) input port.
      mask init:
      | if maskTabDims >= 5
      |   numTDims = explicitNumDims;
      | else
      |   numTDims = maskTabDims;
      | end
      | numInputs =  numTDims - (outDims-1);
      | if tabIsInput == 1
      |   tText = 'T';
      |   tPort = numInputs + 1;
      |   tio   = 'input';
      | else
      |   tText = ' ';
      |   tPort = 1;
      |   tio   = 'output';
      | end
      | if strcmp(get_param(bdroot(gcb),'BlockDiagramType'),'library')
      |   dimsChar = 'n';
      | else
      |   dimsChar = sprintf('%d',numTDims);
      | end
      | [x,y] = nddirectico('plotdata', numTDims, tabIsInput, outDims);
      | xp = x((end-3):end); yp = y((end-3):end);
      | x = x(1:(end-4)); y = y(1:(end-4));
      mask StyleString: popup(1|2|3|4|More...),edit,popup(Element|Column|2-D Matrix),checkbox,edit,popup(None|Warning|Error)
      mask CallbackString: nddirectico('dialog')|||nddirectico('dialog')||
      mask Display:
      | text(0.5,0.9, sprintf(' %s-D T[k]',dimsChar), 'HorizontalAlignment','center')
      | plot(x,y)
      | patch(xp, yp)
      | port_label(tio,tPort,tText)
  Interpolation (n-D) using PreLookup : S-Function  FunctionName=sfun_kflookupnd  Parameters=numDims,table,interpMethod,extrapMethod,rangeErrorMode,NumSelectionDims  mask(LookupNDInterpIdx){numDimsPopupSelect=2, explicitNumDims=2, table=sqrt([1:10]'*[1:10]), interpMethod=Linear, extrapMethod=Linear, rangeErrorMode=None, NumSelectionDims=0}
      mask prompts: numDimsPopupSelect "Number of table dimensions:"; explicitNumDims "Explicit number of table dimensions:"; table "Table data:"; interpMethod "Interpolation method:"; extrapMethod "Extrapolation method:"; rangeErrorMode "Action for out of range input:"; NumSelectionDims "Number of sub-table selection dimensions:"
      mask help: Perform interpolation on an n-dimensional (n-D) table using precalculated indices and distance fractions. An n-D Table is a sampled representation of a function in N variables. This block's 'u' input ports are intended to be fed with the output of a PreLook-Up Index Search block. Interpolation on a selected portion of the table can be optionally performed by specifying how many dimensions are to be used for sub-table selection. Sub-table selection is performed starting with the highest (last) dimension. The 'sel' input ports are fed with a uint32-typed value that is a table index in the corresponding dimension (zero-based indexing). The first dimension input corresponds to the top (or left) input port.
      mask init:
      | if numDimsPopupSelect==5
      |   numDims=explicitNumDims;
      | else
      |   numDims=numDimsPopupSelect;
      | end
      | [x,y,xaxes,yaxes] = ndlookico('plot',numDims, 'LookupNDInterpIdx', table, interpMethod, NumSelectionDims);
      mask StyleString: popup(1|2|3|4|More...),edit,edit,popup(None - Flat|Linear),popup(None - Clip|Linear),popup(None|Warning|Error|Error - No index checking in generated code|Warning - No index checking in generated code|None - No index checking in generated code),edit
      mask CallbackString: ndlookico('kfdyn')||||||
      mask Display:
      | text(0.5,0.9,' n-D T(k,f)','horizontalAlignment','center');
      | plot(x,y);
      | plot(xaxes,yaxes);
  Lookup Table Dynamic : S-Function  FunctionName=sfix_look1_dyn  Parameters=OutputDataTypeScalingMode,(getdatatypespecs(OutDataType,OutScaling,DblOver,0)),[DoSatur RndMeth-1],DblOver,dolog,LookUpMeth  mask(Lookup Table Dynamic){LookUpMeth=Interpolation-Use End Values, OutputDataTypeScalingMode=Specify via dialog, OutDataType=float('double'), OutScaling=2^-10, LockScale=off, RndMeth=Floor, DoSatur=off}
      mask prompts: LookUpMeth "Look-Up Method:"; OutputDataTypeScalingMode "Output data type and scaling:"; OutDataType "Output data type:     ex.  sfix(16),  uint(8),  float('single')"; OutScaling "Output scaling:    Slope or [Slope Bias]    ex.  2^-9"; LockScale "Lock output scaling so autoscaling tool can't change it"; RndMeth "Round toward:"; DoSatur "Saturate to max or min when overflows occur"
      mask help: Approximate a one-dimensional function using a selected look-up method.
      mask init:
      | DblOver = 0;
      | dolog = 0;
      mask StyleString: popup(Interpolation-Extrapolation|Interpolation-Use End Values|Use Input Nearest|Use Input Below|Use Input Above),popup(Specify via dialog|Inherit via back propagation),edit,edit,checkbox,popup(Zero|Nearest|Ceiling|Floor),checkbox
      mask CallbackString: |fixptdialog(gcbh)|fixptdialog(gcbh)||||
      mask TabNameString: Main,Signal data types,Signal data types,Signal data types,Signal data types,Signal data types,Signal data types
      mask Display:
      | port_label('Input',1,'x');
      | port_label('Input',2,'xdat');
      | port_label('Input',3,'ydat');
      | port_label('Output',1,'y');
  Lookup Table (2-D) : Lookup2D  DialogController=Simulink.DDGSource  RowIndex=[1:3]  ColumnIndex=[1:3]  OutputValues=[4 5 6;16 19 20;10 18 23]
  Lookup Table (n-D) : S-Function  FunctionName=sfun_lookupnd  Parameters=numDims,tableData,bp1,bp2,bp3,bp4,bpcell,searchMode,cacheBpFlag,vectorInputFlag,interpMethod,extrapMethod,rangeErrorMode  mask(LookupNDInterp){numDimsPopupSelect=2, bp1=[10,22,31], bp2=[10,22,31], bp3=[1:3], bp4=[1:3], bpcell={ [1:3], [1:3] }, explicitNumDims=2, searchMode=Binary Search, cacheBpFlag=off, vectorInputFlag=off, tableData=[4 5 6;16 19 20;10 18 23], interpMethod=Linear, extrapMethod=Linear, rangeErrorMode=None}
      mask prompts: numDimsPopupSelect "Number of table dimensions:"; bp1 "First input (row) breakpoint set:"; bp2 "Second (column) input breakpoint set:"; bp3 "Third input breakpoint set:"; bp4 "Fourth input breakpoint set:"; bpcell "Fifth..Nth breakpoint sets (cell array):"; explicitNumDims "Explicit number of dimensions:"; searchMode "Index search method:"; cacheBpFlag "Begin index searches using previous index results"; vectorInputFlag "Use one (vector) input port instead of N ports"; tableData "Table data:"; interpMethod "Interpolation method:"; extrapMethod "Extrapolation method:"; rangeErrorMode "Action for out of range input:"
      mask help: Perform n-dimensional interpolated table lookup including index searches. The table is a sampled representation of a function in N variables. Breakpoint sets relate the input values to positions in the table. The first dimension corresponds to the top (or left) input port.
      mask init:
      | if numDimsPopupSelect==5
      |   numDims=explicitNumDims;
      | else
      |   numDims=numDimsPopupSelect;
      | end
      | if strcmp(get_param(bdroot,'BlockDiagramType'),'library')
      |   dimsChar = 'n';
      | else
      |   dimsChar = sprintf('%d',numDims);
      | end
      | switch interpMethod
      |   case 1
      |     plottype = 'flatplot';
      |   case 2
      |     plottype = 'lineplot';
      |   otherwise
      |     plottype = 'splineplot';
      | end
      | 
      | [x,y,xaxes,yaxes] = ndlookico(plottype, numDims, 'LookupNDInterp', tableData, bp1);
      mask StyleString: popup(   1   |   2   |   3   |   4   |More...),edit,edit,edit,edit,edit,edit,popup(Evenly Spaced Points|Linear Search|Binary Search),checkbox,checkbox,edit,popup(None - Flat|Linear|Cubic Spline),popup(None - Clip|Linear|Cubic Spline),popup(None|Warning|Error)
      mask CallbackString: ndlookico|||||||||||||
      mask Display:
      | text(0.5,0.9,sprintf(' %s-D T(u)',dimsChar),'horizontalAlignment','center')
      | plot(x,y)
      | plot(xaxes,yaxes)
  Lookup Table : Lookup  DialogController=Simulink.DDGSource  InputValues=[-5:5]  OutputValues=tanh([-5:5])
  PreLookup Index Search : S-Function  FunctionName=sfun_idxsearch  Parameters=bpData, searchMode, cacheBpFlag, extrapMode, rangeErrorMode, outputFlag, IndexDataType  mask(LookupIdxSearch){bpData=[10:10:100], searchMode=Binary Search, cacheBpFlag=off, outputFlag=off, IndexDataType=uint32, extrapMode=Linear Extrapolation, rangeErrorMode=None}
      mask prompts: bpData "Breakpoint data:"; searchMode "Index search method:"; cacheBpFlag "Begin index search using previous index result"; outputFlag "Output only the index"; IndexDataType "Index data type:"; extrapMode "Process out of range input:"; rangeErrorMode "Action for out of range input:"
      mask help: Locate the input value's relative position within a range of numbers (the "breakpoint data" set). Returns an array of the interval index "k"and distance fraction "f" that the input "u" reaches into the kth interval.
      mask init:
      | if outputFlag == 0
      |   fig = 'f';
      |   f = 'f';
      | else
      |   fig = 'k';
      |   f = '';
      | end
      | [x,y] = ndlookico('bpplotdata', fig);
      | [xp,yp] = ndlookico('bppatchdata');
      mask StyleString: edit,popup(Evenly Spaced Points|Linear Search|Binary Search),checkbox,checkbox,popup(uint32|int32),popup(Clip to Range|Linear Extrapolation),popup(None|Warning|Error)
      mask CallbackString: |||ndlookico('predyn')|||
      mask Display:
      | text(0.13, 0.85, 'u','HorizontalAlignment','center','VerticalAlignment','middle');
      | text(0.4, 0.53, ' k','HorizontalAlignment','center','VerticalAlignment','base');
      | text(0.88, 0.3, f,'HorizontalAlignment','center','VerticalAlignment','middle');
      | plot(x,y);
      | patch(xp, yp);
  Sine : Subsystem  mask(Sine){NumDataPoints=(2^5)+1}
      mask prompts: NumDataPoints "Number of data points for lookup table:"
      mask help:
      | Implement a Sine function in Fixed-Point using a lookup table approach that exploits quarter wave symmetry.  The output is normally a signed 16 bit number with 14 bits to the right of the binary point.
      |
      | The most efficient implementation is obtained when the number of data points is a power of 2 plus 1.  For example, (2^5)+1.
      mask init:
      | XData = linspace(0,0.25,NumDataPoints);
      | YData = sin(2*pi*XData);
      mask Display: disp('sin(2*pi*u)')
  wires:
  PreLookup Index Search/1 -> Interpolation (n-D) using PreLookup/1
